simulink model "sfunctest"  (Simulink 7.9)
settings: Solver=ode45  StartTime=0.0  StopTime=3  MaxStep=0.001  RelTol=1e-3
settings Model: Creator=naa  LastModifiedBy=naa

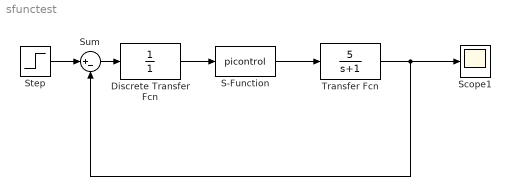
== system sfunctest ==
  Discrete Transfer Fcn : DiscreteTransferFcn  Denominator=[1 ]  SampleTime=0.01
  S-Function : S-Function  FunctionName=picontrol  Parameters="1  0.01"  EnableBusSupport=off
  Scope1 : Scope
  Step : Step  Time=0.1  SampleTime=0
  Sum : Sum  Inputs=|+-
  Transfer Fcn : TransferFcn  Numerator=[5]  Denominator=[1 1]
  wires:
  Step/1 -> Sum/1
  Sum/1 -> Discrete Transfer Fcn/1
  Discrete Transfer Fcn/1 -> S-Function/1
  S-Function/1 -> Transfer Fcn/1
  Transfer Fcn/1 -> Scope1/1, Sum/2
